simulink model "custom_test"  (R2023a)
settings: Solver=FixedStepAuto  StartTime=0.0  StopTime=inf  FixedStep=0.01  RelTol=1e-3  EnableMultiTasking=on
undefined symbols (not defined in the file): dev, Main, pwm_output0
libraries: simulink x4, px4Sensorslib x3, px4lib x1, px4uORBlib x1
settings Model: SimulationMode=external  ExtModeTrigDuration=10  Creator=ArriGE66  LastModifiedBy=User
settings SolverCC: PositivePriorityOrder=on
settings OptimizationCC: EnhancedBackFolding=on  PassReuseOutputArgsAs=Individual arguments  ZeroExternalMemoryAtStartup=off  ZeroInternalMemoryAtStartup=off  MaxStackSize=64  OptimizeBlockOrder=speed  DifferentSizesBufferReuse=on  OptimizationCustomize=off  EfficientTunableParamExpr=on
settings DebuggingCC: ParameterTunabilityLossMsg=error
settings HardwareCC: ProdBitPerPointer=32  ProdBitPerSizeT=32  ProdBitPerPtrDiffT=32  ProdLargestAtomicInteger=Long  ProdLargestAtomicFloat=Double  ProdWordSize=32  ProdLongLongMode=on  ProdHWDeviceType=ARM Compatible->ARM Cortex
settings SFSimCC: MATLABDynamicMemAlloc=off  SimTargetLang=C++
settings RTWCC: Description=Embedded Coder  SystemTargetFile=ert.tlc  HardwareBoard=PX4 Cube Orange  TemplateMakefile=ert_default_tmf  Toolchain=GNU Tools for PX4 Autopilots  TargetLang=C++
settings CodeAppCC: ForceParamTrailComments=on  IgnoreCustomStorageClasses=off  OperatorAnnotations=on  SimulinkDataObjDesc=on  SFDataObjDesc=on  InsertBlockDesc=on
settings ERTTargetCC: ExtMode=on  ExtModeTransport=3  ExtModeStaticAlloc=on  ExtModeStaticAllocSize=1024  ExtModeMexFile=ext_xcp  ExtModeMexArgs=1 COM10 3000000  ExtModeIntrfLevel=Level2 - Open

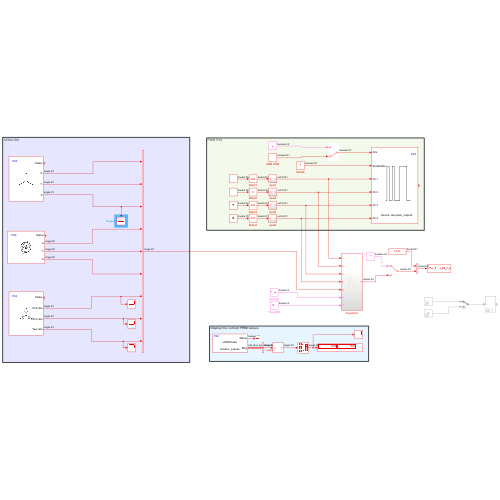
[thumbnail: Simulink's stored preview of the top-level diagram]
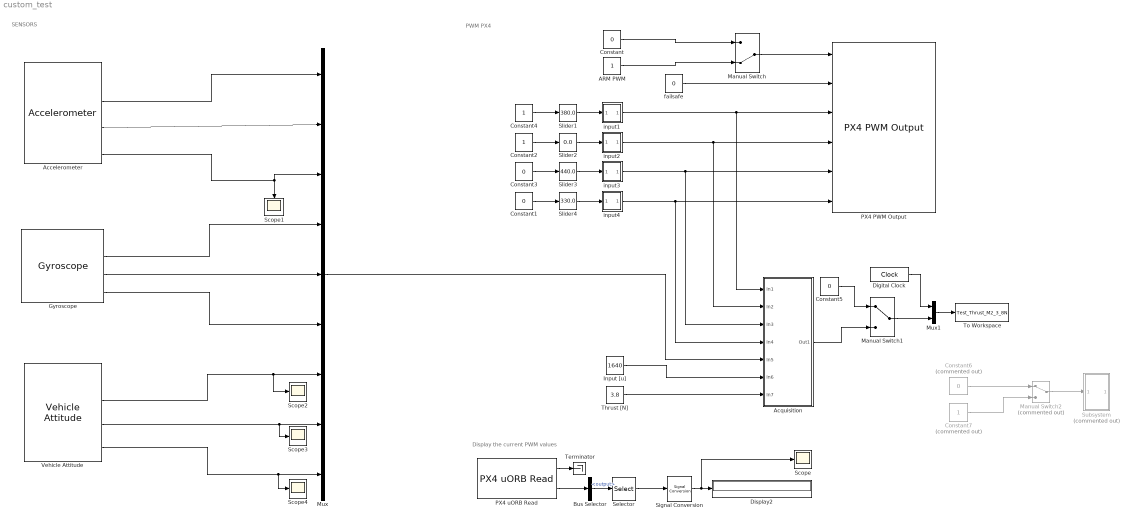
== system custom_test ==
  note: PWM PX4
  note: SENSORS
  note: Display the current PWM values
  ARM PWM : Constant  OutDataTypeStr=boolean  SampleTime=0.01
  Accelerometer : px4Sensorslib/Accelerometer  uorbTimeStamp=off  BlockingMode=off  BlockTimeout=1e-3  sampleTime=1/100
  Acquisition : Subsystem
  Bus Selector : BusSelector  OutputSignals=output
  Constant : Constant  Value=0  OutDataTypeStr=boolean
  Constant1 : Constant  Value=0  SampleTime=0.01
  Constant2 : Constant  SampleTime=0.01
  Constant3 : Constant  Value=0  SampleTime=0.01
  Constant4 : Constant  SampleTime=0.01
  Constant5 : Constant  Value=0  OutDataTypeStr=boolean
  Constant6 : Constant  Commented=on  Value=0
  Constant7 : Constant  Commented=on
  Digital Clock : DigitalClock  SampleTime=-1
  Display2 : Display
  Gyroscope : px4Sensorslib/Gyroscope  uorbTimeStamp=off  BlockingMode=off  BlockTimeout=1e-3  sampleTime=1/100
  Input [u] : Constant  Value=1640  OutDataTypeStr=double
  Manual Switch : ManualSwitch  CurrentSetting=0
  Manual Switch1 : ManualSwitch
  Manual Switch2 : ManualSwitch  Commented=on
  Mux : Mux  Inputs=9
  Mux1 : Mux  Inputs=2
  PX4 PWM Output : px4lib/PX4 PWM Output  pwmDevice=Main (/dev/pwm_output0)  pwmChannel1_=on  pwmChannel2_=on  pwmChannel3_=on  pwmChannel4_=on  pwmChannel5_=off  pwmChannel6_=off  pwmChannel7_=off  pwmChannel8_=off  forceTerminateFailsafe=off  outputErrorStatus=on
  PX4 uORB Read : px4uORBlib/PX4 uORB Read  uORBTopic=actuator_outputs  selectInstance=actuator_outputs  SampleTime=0.01  BlockingMode=off  BlockTimeout=1e-3
  Scope{,1..4} (5 alike) : Scope
  Selector : Selector  InputPortWidth=16  IndexOptions=Index vector (dialog)  Indices=[1 2]  OutputSizes=1
  Signal Conversion : SignalConversion  OverrideOpt=off
  Slider1 : simulink/Math Operations/Slider Gain  gain=380.0  low=0  high=1000
  Slider2 : simulink/Math Operations/Slider Gain  gain=0.0  low=0  high=1000
  Slider3 : simulink/Math Operations/Slider Gain  gain=440.0  low=0  high=1000
  Slider4 : simulink/Math Operations/Slider Gain  gain=330.0  low=0  high=1000
  Subsystem : Subsystem  Commented=on  mask{delta_t=10}
      mask prompts: delta_t "delta_time [s]"
  Terminator : Terminator
  Thrust [N] : Constant  Value=3.8  OutDataTypeStr=double
  To Workspace : ToWorkspace  VariableName=Test_Thrust_M2_3_8N  SampleTime=-1
      settings: Save2DSignal=2-D array (concatenate along first dimension)
  Vehicle Attitude : px4Sensorslib/Vehicle Attitude  rollRate=on  pitchRate=on  yawRate=on  quaternion=off  uorbTimeStamp=off  BlockingMode=off  BlockTimeout=0.001  sampleTime=1/100
  failsafe : Constant  Value=0  OutDataTypeStr=boolean  SampleTime=0.01
  input1 : Subsystem
  input2 : Subsystem
  input3 : Subsystem
  input4 : Subsystem
  wires:
  Manual Switch/1 -> PX4 PWM Output/1
  Bus Selector/1 -> Selector/1  "<output>"
  PX4 uORB Read/1 -> Terminator/1
  failsafe/1 -> PX4 PWM Output/2
  Selector/1 -> Signal Conversion/1
  PX4 uORB Read/2 -> Bus Selector/1
  Signal Conversion/1 -> Scope/1, Display2/1
  Constant1/1 -> Slider4/1
  Slider4/1 -> input4/1(In1)
  Slider2/1 -> input2/1(In1)
  Constant2/1 -> Slider2/1
  Slider3/1 -> input3/1(In1)
  Constant3/1 -> Slider3/1
  Slider1/1 -> input1/1(In1)
  Constant4/1 -> Slider1/1
  input4/1(Out1) -> Acquisition/4(In4), PX4 PWM Output/6
  input3/1(Out1) -> Acquisition/3(In3), PX4 PWM Output/5
  input2/1(Out1) -> Acquisition/2(In2), PX4 PWM Output/4
  input1/1(Out1) -> Acquisition/1(In1), PX4 PWM Output/3
  Vehicle Attitude/3 -> Scope3/1, Mux/8
  Vehicle Attitude/2 -> Scope2/1, Mux/7
  ARM PWM/1 -> Manual Switch/2
  Constant/1 -> Manual Switch/1
  Gyroscope/4 -> Mux/6
  Gyroscope/3 -> Mux/5
  Gyroscope/2 -> Mux/4
  Accelerometer/2 -> Mux/1
  Accelerometer/3 -> Mux/2
  Accelerometer/4 -> Mux/3, Scope1/1
  Mux/1 -> Acquisition/5(In5)
  Input [u]/1 -> Acquisition/6(In6)
  Thrust [N]/1 -> Acquisition/7(In7)
  Acquisition/1(Out1) -> Manual Switch1/2
  Constant5/1 -> Manual Switch1/1
  Mux1/1 -> To Workspace/1
  Digital Clock/1 -> Mux1/1
  Manual Switch1/1 -> Mux1/2
  Constant7/1 -> Manual Switch2/2
  Constant6/1 -> Manual Switch2/1
  Manual Switch2/1 -> Subsystem/1(In1)
  Vehicle Attitude/4 -> Scope4/1, Mux/9

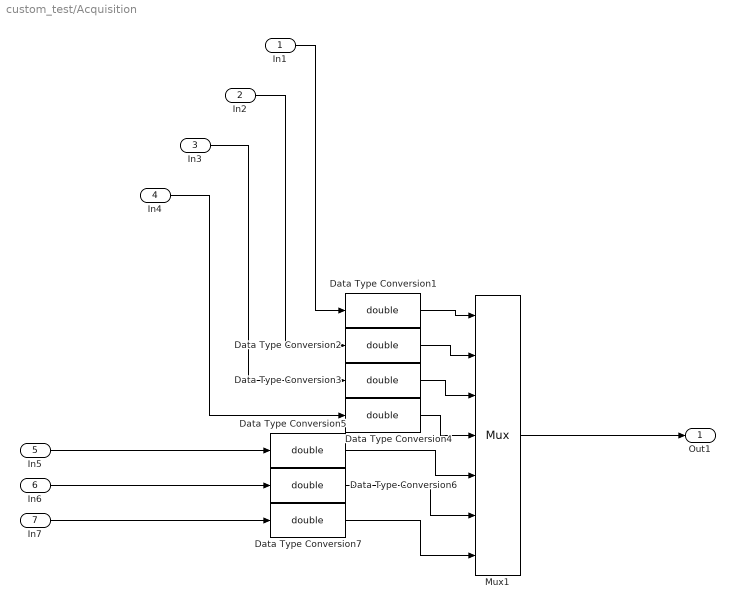
== system custom_test/Acquisition ==
  In1 : Inport
  In2 : Inport  Port=2
  In3 : Inport  Port=3
  In4 : Inport  Port=4
  In5 : Inport  Port=5
  In6 : Inport  Port=6
  In7 : Inport  Port=7
  Data Type Conversion{1..7} (7 alike) : DataTypeConversion  OutDataTypeStr=double  SaturateOnIntegerOverflow=off  RndMeth=Floor
  Mux1 : Mux  Inputs=7
      settings: DisplayOption=signals
  Out1 : Outport
  wires:
  In7/1 -> Data Type Conversion7/1
  In2/1 -> Data Type Conversion2/1
  Data Type Conversion1/1 -> Mux1/1
  Data Type Conversion7/1 -> Mux1/7
  Data Type Conversion3/1 -> Mux1/3
  Data Type Conversion5/1 -> Mux1/5
  Data Type Conversion4/1 -> Mux1/4
  Data Type Conversion2/1 -> Mux1/2
  Data Type Conversion6/1 -> Mux1/6
  In3/1 -> Data Type Conversion3/1
  In6/1 -> Data Type Conversion6/1
  Mux1/1 -> Out1/1
  In5/1 -> Data Type Conversion5/1
  In1/1 -> Data Type Conversion1/1
  In4/1 -> Data Type Conversion4/1

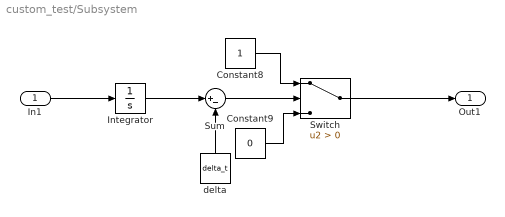
== system custom_test/Subsystem ==
  In1 : Inport
  Constant8 : Constant
  Constant9 : Constant  Value=0
  Integrator : Integrator
  Sum : Sum  Inputs=|+-
  Switch : Switch  Criteria=u2 > Threshold  SaturateOnIntegerOverflow=off  InputSameDT=off
  delta : Constant  Value=delta_t
  Out1 : Outport
  wires:
  delta/1 -> Sum/2
  In1/1 -> Integrator/1
  Sum/1 -> Switch/2
  Integrator/1 -> Sum/1
  Switch/1 -> Out1/1
  Constant9/1 -> Switch/3
  Constant8/1 -> Switch/1

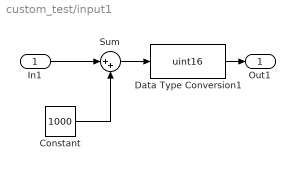
== system custom_test/input1 ==
  In1 : Inport
  Constant : Constant  Value=1000  SampleTime=0.01
  Data Type Conversion1 : DataTypeConversion  OutDataTypeStr=uint16  SaturateOnIntegerOverflow=off  RndMeth=Floor
  Sum : Sum  Inputs=|++
  Out1 : Outport
  wires:
  Sum/1 -> Data Type Conversion1/1
  In1/1 -> Sum/1
  Constant/1 -> Sum/2
  Data Type Conversion1/1 -> Out1/1

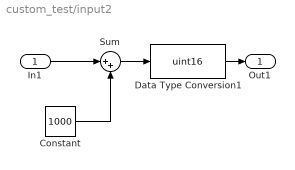
== system custom_test/input2 ==
  In1 : Inport
  Constant : Constant  Value=1000  SampleTime=0.01
  Data Type Conversion1 : DataTypeConversion  OutDataTypeStr=uint16  SaturateOnIntegerOverflow=off  RndMeth=Floor
  Sum : Sum  Inputs=|++
  Out1 : Outport
  wires:
  Sum/1 -> Data Type Conversion1/1
  In1/1 -> Sum/1
  Constant/1 -> Sum/2
  Data Type Conversion1/1 -> Out1/1

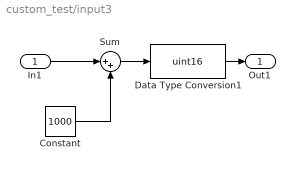
== system custom_test/input3 ==
  In1 : Inport
  Constant : Constant  Value=1000  SampleTime=0.01
  Data Type Conversion1 : DataTypeConversion  OutDataTypeStr=uint16  SaturateOnIntegerOverflow=off  RndMeth=Floor
  Sum : Sum  Inputs=|++
  Out1 : Outport
  wires:
  Sum/1 -> Data Type Conversion1/1
  In1/1 -> Sum/1
  Constant/1 -> Sum/2
  Data Type Conversion1/1 -> Out1/1

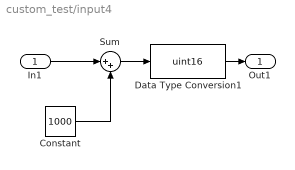
== system custom_test/input4 ==
  In1 : Inport
  Constant : Constant  Value=1000  SampleTime=0.01
  Data Type Conversion1 : DataTypeConversion  OutDataTypeStr=uint16  SaturateOnIntegerOverflow=off  RndMeth=Floor
  Sum : Sum  Inputs=|++
  Out1 : Outport
  wires:
  Sum/1 -> Data Type Conversion1/1
  In1/1 -> Sum/1
  Constant/1 -> Sum/2
  Data Type Conversion1/1 -> Out1/1
